simulink model "Final_Model_Project3"  (R2023b)
settings: Solver=ode23tb  StartTime=0.0  StopTime=2.0  MaxStep=1e-5  RelTol=1e-5  AbsTol=1e-5
values from neighbouring files (symbols this model uses):
  alpha_beta = [1 (-1/2) (-1/2); 0 (sqrt(3)/2) (-sqrt(3)/2)]    [Project3.m]
  DC_Link_Cap = 44571.853e-06    (= 0.044571853)    [Project3.m]
  DC_Link_Res = 30e-03    (= 0.03)    [Project3.m]
  F_sampg = 10000    [Project3.m]
  F_swg = 2040    [Project3.m]
  Fc = 100    [Project3.m]
  Fc1 = 500    [Project3.m]
  Fc2 = 10    [Project3.m]
  Fg = 60    [Project3.m]
  Grid_Filter_Ind = 0.12629e-03    (= 0.00012629)    [Project3.m]
  Grid_Filter_Res = 1.19025e-03    (= 0.00119025)    [Project3.m]
  Grid_Line_RMS_Voltage = 690    [Project3.m]
  I_peak = sqrt(2)*Current_base    [Project3.m]
  L_base_pu = 0.2    [Project3.m]
  P_outapp = 2.00e+06    (= 2000000)    [Project3.m]
  Ref_DC_Voltage = 1220    [Project3.m]
  Ts = 1/F_sampg    (= 0.0001)    [Project3.m]
  V_peak = sqrt(2)*Voltage_base    [Project3.m]
  Voltage_Battery = 1259    [Project3.m]
  w_base_pu = 1    [Project3.m]
libraries: spsVoltageMeasurementLib x5, slpidlib x3, spsSeriesRLCBranchLib x2, simulink x2, spsDCVoltageSourceLib x1, simulink_extras x1, spsThreePhaseSeriesRLCBranchLib x1, spsUniversalBridgeLib x1, spsGroundLib x1, spsThreePhaseProgrammableVoltageSourceLib x1, spsThreePhaseVIMeasurementLib x1, sps_lib x1
settings Model: Creator=priya  LastModifiedBy=priya
settings DataIOCC: ReturnWorkspaceOutputs=off

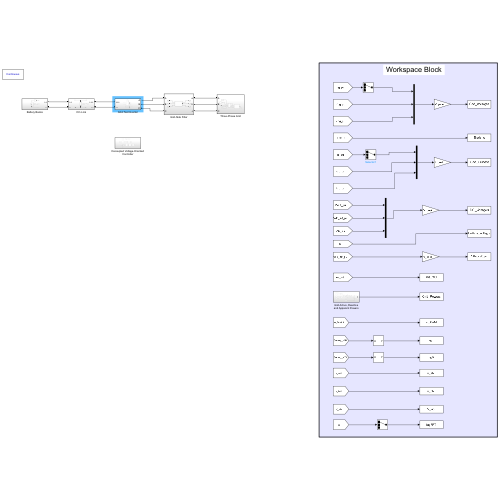
[thumbnail: Simulink's stored preview of the top-level diagram]
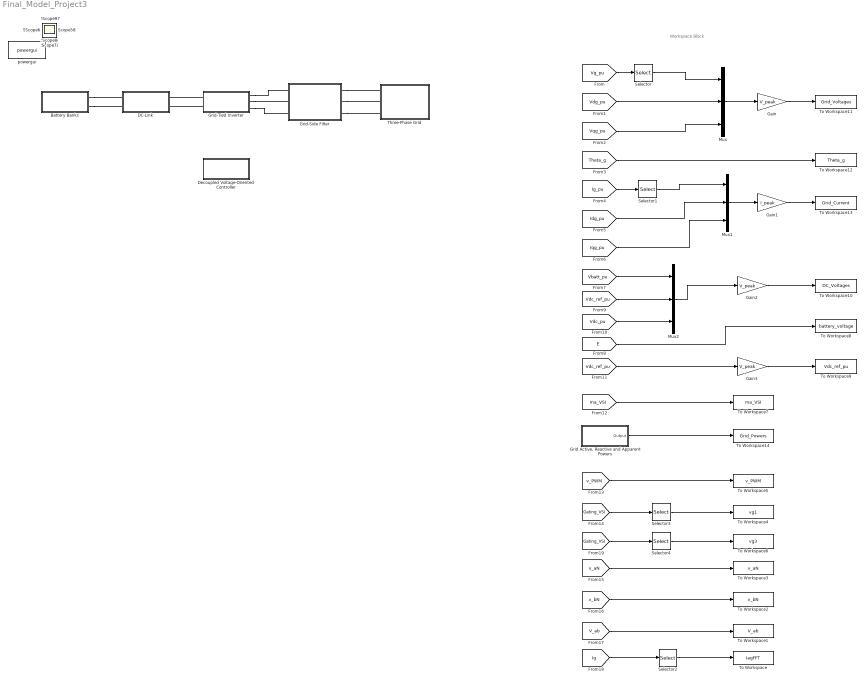
== system Final_Model_Project3 ==
  note: Workspace Block
  Battery Banks : Subsystem
  DC-Link : Subsystem
  Decoupled Voltage-Oriented Controller : Subsystem
  Gain : Gain  Gain=V_peak
  Gain1 : Gain  Gain=I_peak
  Gain2 : Gain  Gain=V_peak
  Gain3 : Gain  Gain=V_peak
  "Grid Active, Reactive and Apparent Powers" : Subsystem
  Grid-Side Filter : Subsystem
  Grid-Tied Inverter : Subsystem
  Mux : Mux  Inputs=3
  Mux1 : Mux  Inputs=3
  Mux2 : Mux  Inputs=3
  Selector : Selector  InputPortWidth=3  IndexOptions=Index vector (dialog)  Indices=[1]  OutputSizes=1
  Selector1 : Selector  InputPortWidth=3  IndexOptions=Index vector (dialog)  Indices=[1]  OutputSizes=1
  Selector2 : Selector  InputPortWidth=3  IndexOptions=Index vector (dialog)  Indices=[1]  OutputSizes=1
  Selector3 : Selector  InputPortWidth=6  IndexOptions=Starting index (dialog)  Indices=[1]  OutputSizes=1
  Selector4 : Selector  InputPortWidth=6  IndexOptions=Starting index (dialog)  Indices=[3]  OutputSizes=1
  Three-Phase Grid : Subsystem
  To Workspace : ToWorkspace  VariableName=IagFFT  SaveFormat=Structure With Time  SampleTime=-1
  To Workspace1 : ToWorkspace  VariableName=V_ab  SampleTime=-1
  To Workspace10 : ToWorkspace  VariableName=DC_Voltages  SampleTime=-1
  To Workspace11 : ToWorkspace  VariableName=Grid_Voltages  SampleTime=-1
  To Workspace12 : ToWorkspace  VariableName=Theta_g  SampleTime=-1
  To Workspace13 : ToWorkspace  VariableName=Grid_Current  SampleTime=-1
  To Workspace14 : ToWorkspace  VariableName=Grid_Powers  SampleTime=-1
  To Workspace2 : ToWorkspace  VariableName=v_bN  SampleTime=-1
  To Workspace3 : ToWorkspace  VariableName=v_aN  SampleTime=-1
  To Workspace4 : ToWorkspace  VariableName=vg1  SampleTime=-1
  To Workspace5 : ToWorkspace  VariableName=v_PWM  SampleTime=-1
  To Workspace6 : ToWorkspace  VariableName=vg3  SampleTime=-1
  To Workspace7 : ToWorkspace  VariableName=ma_VSI  SampleTime=-1
  To Workspace8 : ToWorkspace  VariableName=battery_voltage  SampleTime=-1
  To Workspace9 : ToWorkspace  VariableName=Vdc_ref_pu  SampleTime=-1
  powergui : sps_lib/powergui  Priority=1  SimulationMode=Continuous  SampleTime=50e-6  frequency=60  Iterations=50  frequencyindice=60  Pbase=100e6  ErrMax=1e-4  UnitsV=kV  UnitsW=MW  buscounter=0  FunctionMessages=off  echomessages=off  EnableUseOfTLC=off  CurrentSourceSwitches=off  DisableSnubberDevices=off  DisableRonSwitches=off  DisableVfSwitches=off  DisplayEquations=off  AutomaticDiscreteSolvers=off  SolverType=Tustin/Backward Euler (TBE)  Interpol=off  ExternalGateDelay=off  methode=off  Ts=100  x0status=blocks  SPID=on  SwTol=0  HookPort=off  NonlinearTolerance=1e-4  nMaxIteration=100  ContinueOnMaxIteration=off  RestoreLinks=warning  ResistiveCurrentMeasurement=off  Frange=[0:2:500]  Ylog=off  Xlog=on  ShowGrid=off  save=off  variable=ZData  structure=0  ZoomFFT=off  StartTime=0.0  cycles=1  DisplayStyle=1  fundamental=60  FreqAxis=off  MaxFrequency=1000  frequencyindicesteady=1  RmsSteady=1  display=off
  Scope{,1..10,14..19} (17 alike) : Scope
  wires:
  [Vg_pu] -> Selector/1
  [Ig_pu] -> Selector1/1
  Selector/1 -> Mux/1
  [Vdg_pu] -> Mux/2
  [Vqg_pu] -> Mux/3
  Selector1/1 -> Mux1/1
  [Idg_pu] -> Mux1/2
  [Iqg_pu] -> Mux1/3
  Mux/1 -> Gain/1
  Mux1/1 -> Gain1/1
  [E] -> To Workspace8/1
  [Vbatt_pu] -> Mux2/1
  [Vdc_ref_pu] -> Mux2/2
  [Vdc_pu] -> Mux2/3
  Mux2/1 -> Gain2/1
  [Vdc_ref_pu] -> Gain3/1
  [Ig] -> Selector2/1
  Selector2/1 -> To Workspace/1
  [V_ab] -> To Workspace1/1
  [v_bN] -> To Workspace2/1
  [v_aN] -> To Workspace3/1
  [v_PWM] -> To Workspace5/1
  [Gating_VSI] -> Selector3/1
  Selector3/1 -> To Workspace4/1
  [Gating_VSI] -> Selector4/1
  Selector4/1 -> To Workspace6/1
  [ma_VSI] -> To Workspace7/1
  Gain3/1 -> To Workspace9/1
  Gain2/1 -> To Workspace10/1
  Gain/1 -> To Workspace11/1
  [Theta_g] -> To Workspace12/1
  Gain1/1 -> To Workspace13/1
  "Grid Active, Reactive and Apparent Powers"/1(Output) -> To Workspace14/1
  connections:
  Battery Banks/LConn1 -- DC-Link/LConn1
  Battery Banks/LConn2 -- DC-Link/LConn2
  Grid-Side Filter/RConn1 -- Three-Phase Grid/LConn1
  Grid-Side Filter/RConn2 -- Three-Phase Grid/LConn2
  Grid-Side Filter/RConn3 -- Three-Phase Grid/LConn3
  Grid-Tied Inverter/LConn1 -- DC-Link/RConn1
  Grid-Tied Inverter/LConn2 -- DC-Link/RConn2
  Grid-Tied Inverter/RConn1 -- Grid-Side Filter/LConn1
  Grid-Tied Inverter/RConn2 -- Grid-Side Filter/LConn2
  Grid-Tied Inverter/RConn3 -- Grid-Side Filter/LConn3

== system Final_Model_Project3/Battery Banks ==
  DC Voltage Source : spsDCVoltageSourceLib/DC Voltage Source  Amplitude=Voltage_Battery  Measurements=None
  Series RLC Branch : spsSeriesRLCBranchLib/Series RLC Branch  LConnTagsString=__new0  RConnTagsString=__new0  BranchType=R  Resistance=DC_Link_Res  Inductance=1e-3  SetiL0=off  InitialCurrent=0  Capacitance=1e-6  Setx0=off  InitialVoltage=0  Measurements=None
  Voltage Measurement : spsVoltageMeasurementLib/Voltage Measurement  PhasorSimulation=off  OutputType=Complex  PSBequivalent=0
  ++ : PMIOPort  Side=Left
  -- : PMIOPort  Port=2  Side=Left
  tag scope: E=global
  wires:
  Voltage Measurement/1 -> [E]
  connections:
  --/RConn1 -- Voltage Measurement/LConn2 -- DC Voltage Source/LConn1
  Voltage Measurement/LConn1 -- Series RLC Branch/LConn1 -- DC Voltage Source/RConn1
  Series RLC Branch/RConn1 -- ++/RConn1

== system Final_Model_Project3/DC-Link ==
  Cdc : spsSeriesRLCBranchLib/Series RLC Branch  LConnTagsString=__new0  RConnTagsString=__new0  BranchType=C  Resistance=1  Inductance=1e-3  SetiL0=off  InitialCurrent=0  Capacitance=DC_Link_Cap  Setx0=on  InitialVoltage=2*Ref_DC_Voltage  Measurements=None
  Voltage Measurement : spsVoltageMeasurementLib/Voltage Measurement  PhasorSimulation=off  OutputType=Complex  PSBequivalent=0
  ++ : PMIOPort  Side=Left
  -- : PMIOPort  Port=2  Side=Left
  +++ : PMIOPort  Port=3  Side=Right
  --- : PMIOPort  Port=4  Side=Right
  tag scope: Vdc=global
  wires:
  Voltage Measurement/1 -> [Vdc]
  connections:
  Cdc/LConn1 -- Voltage Measurement/LConn1 -- ++/RConn1 -- +++/RConn1
  Cdc/RConn1 -- Voltage Measurement/LConn2 -- --/RConn1 -- ---/RConn1

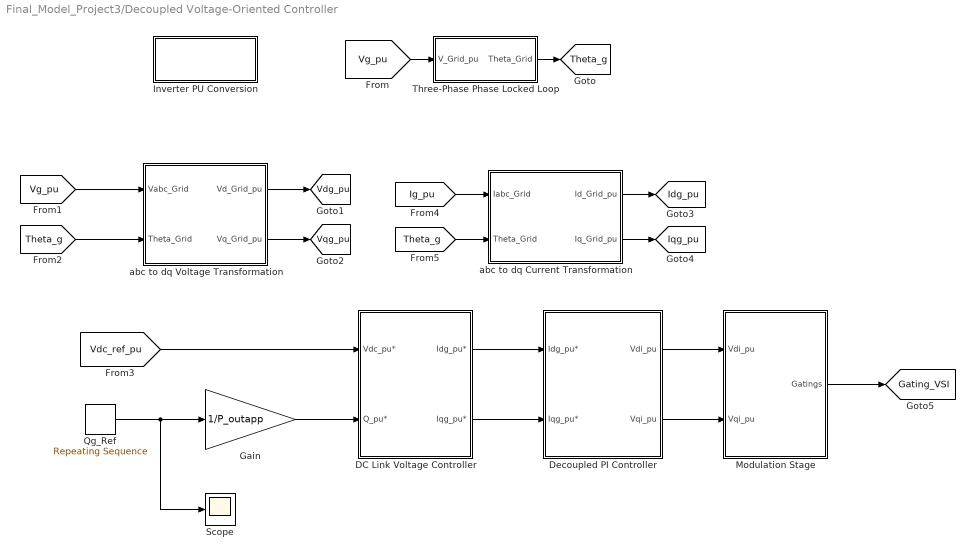
== system Final_Model_Project3/Decoupled Voltage-Oriented Controller ==
  DC Link Voltage Controller : Subsystem
  Decoupled PI Controller : Subsystem
  Gain : Gain  Gain=1/P_outapp
  Inverter PU Conversion : Subsystem
  Modulation Stage : Subsystem
  Qg_Ref : simulink/Sources/Repeating Sequence  rep_seq_t=[0 0.4 0.6 0.8 1 1.2 1.4 1.6 1.8 2]  rep_seq_y=[0 0 1.2e6 1.2e6 0 0 -0.7749e6 -0.7749e6 0 0]
  Scope : Scope
  Three-Phase Phase Locked Loop : Subsystem
  abc to dq Current Transformation : Subsystem
  abc to dq Voltage Transformation : Subsystem
  tag scope: Gating_VSI=global, Idg_pu=global, Iqg_pu=global, Theta_g=global, Vdg_pu=global, Vqg_pu=global
  wires:
  [Vg_pu] -> Three-Phase Phase Locked Loop/1(V_Grid_pu)
  Three-Phase Phase Locked Loop/1(Theta_Grid) -> [Theta_g]
  [Vg_pu] -> abc to dq Voltage Transformation/1(Vabc_Grid)
  [Theta_g] -> abc to dq Voltage Transformation/2(Theta_Grid)
  abc to dq Voltage Transformation/1(Vd_Grid_pu) -> [Vdg_pu]
  abc to dq Voltage Transformation/2(Vq_Grid_pu) -> [Vqg_pu]
  Qg_Ref/1 -> Scope/1, Gain/1
  [Vdc_ref_pu] -> DC Link Voltage Controller/1(Vdc_pu*)
  Gain/1 -> DC Link Voltage Controller/2(Q_pu*)
  [Ig_pu] -> abc to dq Current Transformation/1(Iabc_Grid)
  [Theta_g] -> abc to dq Current Transformation/2(Theta_Grid)
  abc to dq Current Transformation/1(Id_Grid_pu) -> [Idg_pu]
  abc to dq Current Transformation/2(Iq_Grid_pu) -> [Iqg_pu]
  DC Link Voltage Controller/1(Idg_pu*) -> Decoupled PI Controller/1(Idg_pu*)
  DC Link Voltage Controller/2(Iqg_pu*) -> Decoupled PI Controller/2(Iqg_pu*)
  Decoupled PI Controller/1(Vdi_pu) -> Modulation Stage/1(Vdi_pu)
  Decoupled PI Controller/2(Vqi_pu) -> Modulation Stage/2(Vqi_pu)
  Modulation Stage/1(Gatings) -> [Gating_VSI]

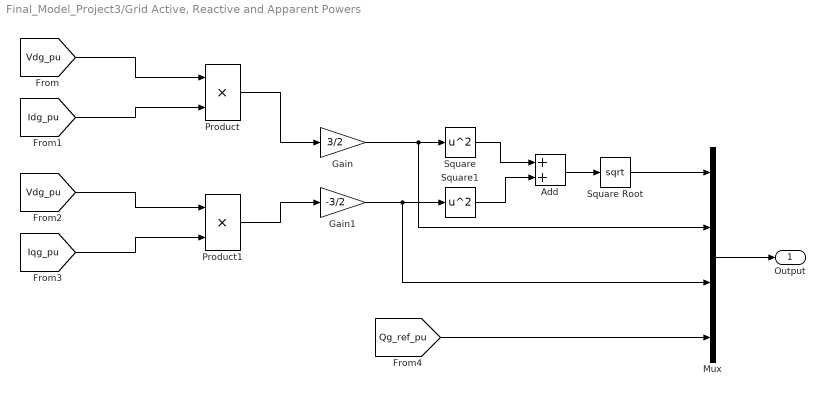
== system Final_Model_Project3/Grid Active, Reactive and Apparent Powers ==
  Add : Sum
  Gain : Gain  Gain=3/2
  Gain1 : Gain  Gain=-3/2
  Mux : Mux
  Product : Product
  Product1 : Product
  Square : Math  Operator=square
  Square Root : Sqrt
  Square1 : Math  Operator=square
  Output : Outport
  wires:
  [Vdg_pu] -> Product/1
  [Idg_pu] -> Product/2
  Product/1 -> Gain/1
  [Vdg_pu] -> Product1/1
  [Iqg_pu] -> Product1/2
  Product1/1 -> Gain1/1
  Gain/1 -> Mux/2, Square/1
  Gain1/1 -> Mux/3, Square1/1
  Square/1 -> Add/1
  Square1/1 -> Add/2
  Add/1 -> Square Root/1
  Square Root/1 -> Mux/1
  [Qg_ref_pu] -> Mux/4
  Mux/1 -> Output/1

== system Final_Model_Project3/Grid-Side Filter ==
  Three-Phase Series RLC Branch : spsThreePhaseSeriesRLCBranchLib/Three-Phase Series RLC Branch  LConnTagsString=A|B|C  RConnTagsString=A|B|C  BranchType=RL  Resistance=Grid_Filter_Res  Inductance=Grid_Filter_Ind  Capacitance=1e-6  Measurements=None
  A : PMIOPort  Side=Left
  B : PMIOPort  Port=2  Side=Left
  C : PMIOPort  Port=3  Side=Left
  a : PMIOPort  Port=4  Side=Right
  b : PMIOPort  Port=5  Side=Right
  c : PMIOPort  Port=6  Side=Right
  connections:
  Three-Phase Series RLC Branch/LConn1 -- a/RConn1
  Three-Phase Series RLC Branch/LConn2 -- b/RConn1
  c/RConn1 -- Three-Phase Series RLC Branch/LConn3
  A/RConn1 -- Three-Phase Series RLC Branch/RConn1
  B/RConn1 -- Three-Phase Series RLC Branch/RConn2
  C/RConn1 -- Three-Phase Series RLC Branch/RConn3

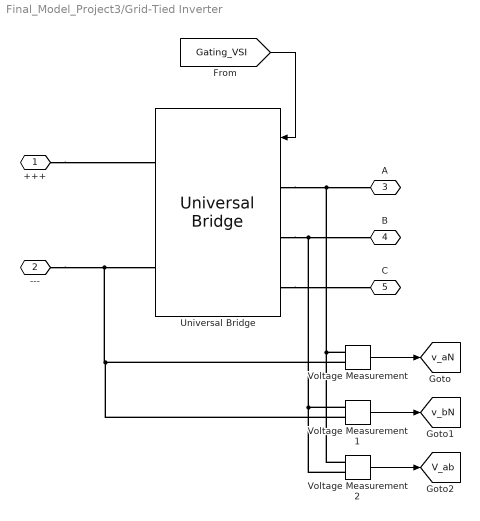
== system Final_Model_Project3/Grid-Tied Inverter ==
  Universal Bridge : spsUniversalBridgeLib/Universal Bridge  Arms=3  SnubberResistance=1e5  SnubberCapacitance=inf  Device=IGBT / Diodes  Ron=1e-6  Lon=0  ForwardVoltages="[  0  0  ]"  ForwardVoltage=0  GTOparameters=[ 10e-6 , 20e-6 ]  IGBTparameters=[ 1e-6 , 2e-6 ]  Measurements=None  Measurements_2=None  converterType=Rectifier
  Voltage Measurement : spsVoltageMeasurementLib/Voltage Measurement  PhasorSimulation=off  OutputType=Complex  PSBequivalent=0
  Voltage Measurement1 : spsVoltageMeasurementLib/Voltage Measurement  PhasorSimulation=off  OutputType=Complex  PSBequivalent=0
  Voltage Measurement2 : spsVoltageMeasurementLib/Voltage Measurement  PhasorSimulation=off  OutputType=Complex  PSBequivalent=0
  +++ : PMIOPort  Side=Left
  --- : PMIOPort  Port=2  Side=Left
  A : PMIOPort  Port=3  Side=Right
  B : PMIOPort  Port=4  Side=Right
  C : PMIOPort  Port=5  Side=Right
  tag scope: V_ab=global, v_aN=global, v_bN=global
  wires:
  [Gating_VSI] -> Universal Bridge/1
  Voltage Measurement/1 -> [v_aN]
  Voltage Measurement1/1 -> [v_bN]
  Voltage Measurement2/1 -> [V_ab]
  connections:
  +++/RConn1 -- Universal Bridge/RConn1
  ---/RConn1 -- Voltage Measurement1/LConn2 -- Voltage Measurement/LConn2 -- Universal Bridge/RConn2
  Universal Bridge/LConn1 -- Voltage Measurement2/LConn1 -- Voltage Measurement/LConn1 -- A/RConn1
  Universal Bridge/LConn2 -- Voltage Measurement2/LConn2 -- Voltage Measurement1/LConn1 -- B/RConn1
  Universal Bridge/LConn3 -- C/RConn1

== system Final_Model_Project3/Three-Phase Grid ==
  Ground : spsGroundLib/Ground  LConnTagsString=a
  Three-Phase Programmable Voltage Source : spsThreePhaseProgrammableVoltageSourceLib/Three-Phase Programmable Voltage Source  PositiveSequence=[Grid_Line_RMS_Voltage 0 Fg]  VariationEntity=None  VariationType=Table of time-amplitude pairs  VariationTypeAlt=Step  VariationStep=0.5  VariationRate=10  VariationMagnitude=0.3  VariationFrequency=2  VariationTiming=[1 2]  VariationPhaseA=off  Amplitudes=[1 0.8 1.2 1.0]  TimeValues=[0 0.1 0.15 0.2]  HarmonicGeneration=off  HarmonicA=[3 0.2 -25 0]  HarmonicB=[2 0.15 35 2]  Timing="[0.05  3]"  BusType=swing  Pref=0  Qref=0  Qmin=-inf  Qmax=inf
  Three-Phase V-I Measurement : spsThreePhaseVIMeasurementLib/Three-Phase V-I Measurement  VoltageMeasurement=phase-to-ground  SetLabelV=off  LabelV=Vabc  Vpu=off  VpuLL=off  CurrentMeasurement=yes  SetLabelI=off  LabelI=Iabc  Ipu=off  Pbase=100e6  Vbase=500e3  OutputType=Complex  PhasorSimulation=off  PSBequivalent=0
  A : PMIOPort  Side=Left
  B : PMIOPort  Port=2  Side=Left
  C : PMIOPort  Port=3  Side=Left
  tag scope: Ig=global, Vg=global
  wires:
  Three-Phase V-I Measurement/1 -> [Vg]
  Three-Phase V-I Measurement/2 -> [Ig]
  connections:
  Three-Phase Programmable Voltage Source/LConn1 -- Ground/LConn1
  Three-Phase V-I Measurement/LConn1 -- Three-Phase Programmable Voltage Source/RConn1
  Three-Phase V-I Measurement/LConn2 -- Three-Phase Programmable Voltage Source/RConn2
  Three-Phase V-I Measurement/LConn3 -- Three-Phase Programmable Voltage Source/RConn3
  Three-Phase V-I Measurement/RConn1 -- A/RConn1
  Three-Phase V-I Measurement/RConn2 -- B/RConn1
  Three-Phase V-I Measurement/RConn3 -- C/RConn1

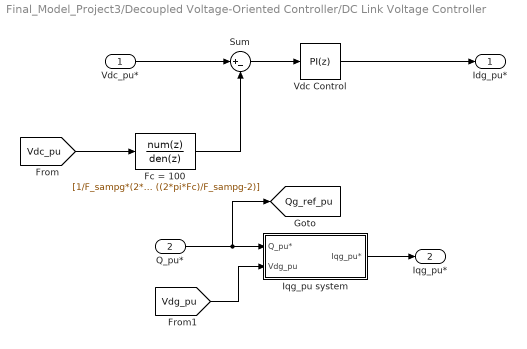
== system Final_Model_Project3/Decoupled Voltage-Oriented Controller/DC Link Voltage Controller ==
  Vdc_pu* : Inport
  Q_pu* : Inport  Port=2
  Fc = 100 : DiscreteTransferFcn  Numerator=[1/F_sampg*(2*pi*Fc) 1/F_sampg*(2*pi*Fc)]  Denominator=[((2*pi*Fc)/F_sampg+2) ((2*pi*Fc)/F_sampg-2)]  SampleTime=Ts
  Iqg_pu system : Subsystem
  Sum : Sum  Inputs=|+-
  Vdc Control : slpidlib/PID Controller  Controller=PI  Form=Parallel  TimeDomain=Discrete-time  UseExternalTs=off  SampleTime=Ts  IntegratorMethod=Forward Euler  FilterMethod=Forward Euler  ControllerParametersSource=internal  P=1  I=200  UseKiTs=off  D=0  N=100  UseFilter=on  TunerSelectOption=Transfer Function Based (PID Tuner App)  InitialConditionSource=internal  InitialConditionForIntegrator=0  InitialConditionForFilter=0  DifferentiatorICPrevScaledInput=0  ExternalReset=none  TrackingMode=off  Kt=1  LimitOutput=on  SatLimitsSource=internal  UpperSaturationLimit=1.5  LowerSaturationLimit=-1.5  LinearizeAsGain=on  AntiWindupMode=none  Kb=1  LimitIntegrator=off  UpperIntegratorSaturationLimit=inf  LowerIntegratorSaturationLimit=-inf  POutMin=[]  POutMax=[]  IOutMin=[]  IOutMax=[]  DOutMin=[]  DOutMax=[]  NOutMin=[]  NOutMax=[]  SumOutMin=[]  SumOutMax=[]  SaturationOutMin=[]  SaturationOutMax=[]  PParamMin=[]  PParamMax=[]  IParamMin=[]  IParamMax=[]  DParamMin=[]  DParamMax=[]  NParamMin=[]  NParamMax=[]  KbParamMin=[]  KbParamMax=[]  KtParamMin=[]  KtParamMax=[]  KbOutMin=[]  KbOutMax=[]  KtOutMin=[]  KtOutMax=[]  IntegratorOutMin=[]  IntegratorOutMax=[]  FilterOutMin=[]  FilterOutMax=[]  SumI1OutMin=[]  SumI1OutMax=[]  SumI2OutMin=[]  SumI2OutMax=[]  SumI3OutMin=[]  SumI3OutMax=[]  SumI4OutMin=[]  SumI4OutMax=[]  SumDOutMin=[]  SumDOutMax=[]  DifferentiatorOutMin=[]  DifferentiatorOutMax=[]  FilterDiffOutCoefMin=[]  FilterDiffOutCoefMax=[]  ReciprocalOutMin=[]  ReciprocalOutMax=[]  SumDenOutMin=[]  SumDenOutMax=[]  SumNumOutMin=[]  SumNumOutMax=[]  DivideOutMin=[]  DivideOutMax=[]  UdiffTsProdOutMin=[]  UdiffTsProdOutMax=[]  NTsProdOutMin=[]  NTsProdOutMax=[]  UintegralTsProdOutMin=[]  UintegralTsProdOutMax=[]  UngainTsProdOutMin=[]  UngainTsProdOutMax=[]  ClampingZeroOutDataTypeStr=Inherit: Inherit via back propagation  ClampingZeroOutMin=[]  ClampingZeroOutMax=[]  FilterDenConstantOutDataTypeStr=Inherit: Inherit via back propagation  FilterDenConstantOutMin=[]  FilterDenConstantOutMax=[]  PCopyOutDataTypeStr=Inherit: Inherit via back propagation  PCopyOutMin=[]  PCopyOutMax=[]  NCopyOutDataTypeStr=Inherit: Inherit via back propagation  NCopyOutMin=[]  NCopyOutMax=[]  IntegratorContinuousStateAttributes=''  IntegratorStateMustResolveToSignalObject=off  IntegratorRTWStateStorageClass=Auto  FilterContinuousStateAttributes=''  FilterStateMustResolveToSignalObject=off  FilterRTWStateStorageClass=Auto  ParallelPVariant=InternalParameters  IdealPVariant=Disabled  IVariant=InternalParameters  DVariant=Disabled  IntegratorVariant=Discrete  SatVariant=Enabled  AWVariant=Passthrough  PCopyVariant=Disabled  TRVariant=Disabled  FdbkBlocksVariant=Forward  IdealPFdbkVariant=Disabled  SatFdbkVariant=Disabled  DerivativeFilterVariant=Disabled  NVariant=Disabled  NCopyVariant=Disabled_SignalSpec  FilterICVariant=Disabled  IntegratorICVariant=InternalICs  ExternalResetVariant=Disabled  TRSumVariant=Passthrough  SumFdbkVariant=Disabled  SumVariant=Sum_PI  TsampFilterVariant=InternalTs  TsampNgainVariant=Passthrough  TsampIntegralVariant=Disabled_SignalSpec  ExternalSaturationOutDataTypeStr=Inherit: Same as second input
  Idg_pu* : Outport
  Iqg_pu* : Outport  Port=2
  tag scope: Qg_ref_pu=global
  wires:
  Vdc_pu*/1 -> Sum/1
  Fc = 100/1 -> Sum/2
  Q_pu*/1 -> [Qg_ref_pu], Iqg_pu system/1(Q_pu*)
  [Vdg_pu] -> Iqg_pu system/2(Vdg_pu)
  Iqg_pu system/1(Iqg_pu*) -> Iqg_pu*/1
  [Vdc_pu] -> Fc = 100/1
  Sum/1 -> Vdc Control/1
  Vdc Control/1 -> Idg_pu*/1

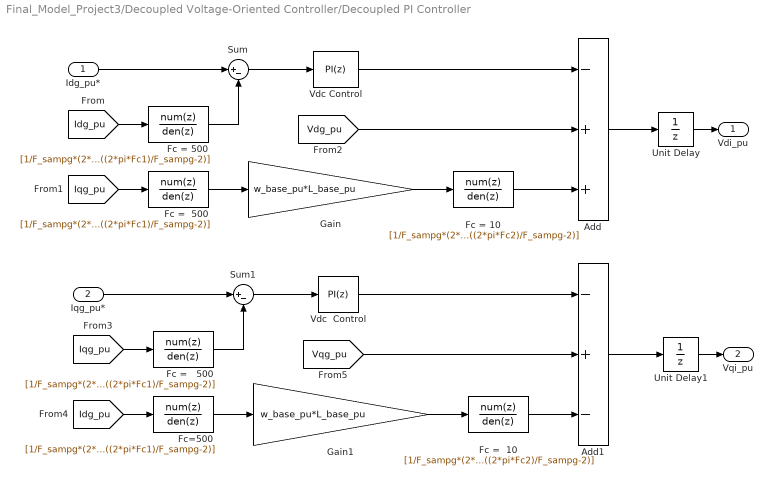
== system Final_Model_Project3/Decoupled Voltage-Oriented Controller/Decoupled PI Controller ==
  Idg_pu* : Inport
  Iqg_pu* : Inport  Port=2
  Add : Sum  Inputs=-++
  Add1 : Sum  Inputs=-+-
  Fc =   500 : DiscreteTransferFcn  Numerator=[1/F_sampg*(2*pi*Fc1) 1/F_sampg*(2*pi*Fc1)]  Denominator=[((2*pi*Fc1)/F_sampg+2) ((2*pi*Fc1)/F_sampg-2)]  SampleTime=Ts
  Fc =  10 : DiscreteTransferFcn  Numerator=[1/F_sampg*(2*pi*Fc2) 1/F_sampg*(2*pi*Fc2)]  Denominator=[((2*pi*Fc2)/F_sampg+2) ((2*pi*Fc2)/F_sampg-2)]  SampleTime=Ts
  Fc =  500 : DiscreteTransferFcn  Numerator=[1/F_sampg*(2*pi*Fc1) 1/F_sampg*(2*pi*Fc1)]  Denominator=[((2*pi*Fc1)/F_sampg+2) ((2*pi*Fc1)/F_sampg-2)]  SampleTime=Ts
  Fc = 10 : DiscreteTransferFcn  Numerator=[1/F_sampg*(2*pi*Fc2) 1/F_sampg*(2*pi*Fc2)]  Denominator=[((2*pi*Fc2)/F_sampg+2) ((2*pi*Fc2)/F_sampg-2)]  SampleTime=Ts
  Fc = 500 : DiscreteTransferFcn  Numerator=[1/F_sampg*(2*pi*Fc1) 1/F_sampg*(2*pi*Fc1)]  Denominator=[((2*pi*Fc1)/F_sampg+2) ((2*pi*Fc1)/F_sampg-2)]  SampleTime=Ts
  Fc=500 : DiscreteTransferFcn  Numerator=[1/F_sampg*(2*pi*Fc1) 1/F_sampg*(2*pi*Fc1)]  Denominator=[((2*pi*Fc1)/F_sampg+2) ((2*pi*Fc1)/F_sampg-2)]  SampleTime=Ts
  Gain : Gain  Gain=w_base_pu*L_base_pu
  Gain1 : Gain  Gain=w_base_pu*L_base_pu
  Sum : Sum  Inputs=|+-
  Sum1 : Sum  Inputs=|+-
  Unit Delay : UnitDelay  SampleTime=Ts  HasFrameUpgradeWarning=on
  Unit Delay1 : UnitDelay  SampleTime=Ts  HasFrameUpgradeWarning=on
  Vdc  Control : slpidlib/PID Controller  Controller=PI  Form=Parallel  TimeDomain=Discrete-time  UseExternalTs=off  SampleTime=Ts  IntegratorMethod=Forward Euler  FilterMethod=Forward Euler  ControllerParametersSource=internal  P=0.3  I=200  UseKiTs=off  D=0  N=100  UseFilter=on  TunerSelectOption=Transfer Function Based (PID Tuner App)  InitialConditionSource=internal  InitialConditionForIntegrator=0  InitialConditionForFilter=0  DifferentiatorICPrevScaledInput=0  ExternalReset=none  TrackingMode=off  Kt=1  LimitOutput=on  SatLimitsSource=internal  UpperSaturationLimit=1.0  LowerSaturationLimit=-1.0  LinearizeAsGain=on  AntiWindupMode=none  Kb=1  LimitIntegrator=off  UpperIntegratorSaturationLimit=inf  LowerIntegratorSaturationLimit=-inf  POutMin=[]  POutMax=[]  IOutMin=[]  IOutMax=[]  DOutMin=[]  DOutMax=[]  NOutMin=[]  NOutMax=[]  SumOutMin=[]  SumOutMax=[]  SaturationOutMin=[]  SaturationOutMax=[]  PParamMin=[]  PParamMax=[]  IParamMin=[]  IParamMax=[]  DParamMin=[]  DParamMax=[]  NParamMin=[]  NParamMax=[]  KbParamMin=[]  KbParamMax=[]  KtParamMin=[]  KtParamMax=[]  KbOutMin=[]  KbOutMax=[]  KtOutMin=[]  KtOutMax=[]  IntegratorOutMin=[]  IntegratorOutMax=[]  FilterOutMin=[]  FilterOutMax=[]  SumI1OutMin=[]  SumI1OutMax=[]  SumI2OutMin=[]  SumI2OutMax=[]  SumI3OutMin=[]  SumI3OutMax=[]  SumI4OutMin=[]  SumI4OutMax=[]  SumDOutMin=[]  SumDOutMax=[]  DifferentiatorOutMin=[]  DifferentiatorOutMax=[]  FilterDiffOutCoefMin=[]  FilterDiffOutCoefMax=[]  ReciprocalOutMin=[]  ReciprocalOutMax=[]  SumDenOutMin=[]  SumDenOutMax=[]  SumNumOutMin=[]  SumNumOutMax=[]  DivideOutMin=[]  DivideOutMax=[]  UdiffTsProdOutMin=[]  UdiffTsProdOutMax=[]  NTsProdOutMin=[]  NTsProdOutMax=[]  UintegralTsProdOutMin=[]  UintegralTsProdOutMax=[]  UngainTsProdOutMin=[]  UngainTsProdOutMax=[]  ClampingZeroOutDataTypeStr=Inherit: Inherit via back propagation  ClampingZeroOutMin=[]  ClampingZeroOutMax=[]  FilterDenConstantOutDataTypeStr=Inherit: Inherit via back propagation  FilterDenConstantOutMin=[]  FilterDenConstantOutMax=[]  PCopyOutDataTypeStr=Inherit: Inherit via back propagation  PCopyOutMin=[]  PCopyOutMax=[]  NCopyOutDataTypeStr=Inherit: Inherit via back propagation  NCopyOutMin=[]  NCopyOutMax=[]  IntegratorContinuousStateAttributes=''  IntegratorStateMustResolveToSignalObject=off  IntegratorRTWStateStorageClass=Auto  FilterContinuousStateAttributes=''  FilterStateMustResolveToSignalObject=off  FilterRTWStateStorageClass=Auto  ParallelPVariant=InternalParameters  IdealPVariant=Disabled  IVariant=InternalParameters  DVariant=Disabled  IntegratorVariant=Discrete  SatVariant=Enabled  AWVariant=Passthrough  PCopyVariant=Disabled  TRVariant=Disabled  FdbkBlocksVariant=Forward  IdealPFdbkVariant=Disabled  SatFdbkVariant=Disabled  DerivativeFilterVariant=Disabled  NVariant=Disabled  NCopyVariant=Disabled_SignalSpec  FilterICVariant=Disabled  IntegratorICVariant=InternalICs  ExternalResetVariant=Disabled  TRSumVariant=Passthrough  SumFdbkVariant=Disabled  SumVariant=Sum_PI  TsampFilterVariant=InternalTs  TsampNgainVariant=Passthrough  TsampIntegralVariant=Disabled_SignalSpec  ExternalSaturationOutDataTypeStr=Inherit: Same as second input
  Vdc Control : slpidlib/PID Controller  Controller=PI  Form=Parallel  TimeDomain=Discrete-time  UseExternalTs=off  SampleTime=Ts  IntegratorMethod=Forward Euler  FilterMethod=Forward Euler  ControllerParametersSource=internal  P=0.3  I=200  UseKiTs=off  D=0  N=100  UseFilter=on  TunerSelectOption=Transfer Function Based (PID Tuner App)  InitialConditionSource=internal  InitialConditionForIntegrator=0  InitialConditionForFilter=0  DifferentiatorICPrevScaledInput=0  ExternalReset=none  TrackingMode=off  Kt=1  LimitOutput=on  SatLimitsSource=internal  UpperSaturationLimit=1.0  LowerSaturationLimit=-1.0  LinearizeAsGain=on  AntiWindupMode=none  Kb=1  LimitIntegrator=off  UpperIntegratorSaturationLimit=inf  LowerIntegratorSaturationLimit=-inf  POutMin=[]  POutMax=[]  IOutMin=[]  IOutMax=[]  DOutMin=[]  DOutMax=[]  NOutMin=[]  NOutMax=[]  SumOutMin=[]  SumOutMax=[]  SaturationOutMin=[]  SaturationOutMax=[]  PParamMin=[]  PParamMax=[]  IParamMin=[]  IParamMax=[]  DParamMin=[]  DParamMax=[]  NParamMin=[]  NParamMax=[]  KbParamMin=[]  KbParamMax=[]  KtParamMin=[]  KtParamMax=[]  KbOutMin=[]  KbOutMax=[]  KtOutMin=[]  KtOutMax=[]  IntegratorOutMin=[]  IntegratorOutMax=[]  FilterOutMin=[]  FilterOutMax=[]  SumI1OutMin=[]  SumI1OutMax=[]  SumI2OutMin=[]  SumI2OutMax=[]  SumI3OutMin=[]  SumI3OutMax=[]  SumI4OutMin=[]  SumI4OutMax=[]  SumDOutMin=[]  SumDOutMax=[]  DifferentiatorOutMin=[]  DifferentiatorOutMax=[]  FilterDiffOutCoefMin=[]  FilterDiffOutCoefMax=[]  ReciprocalOutMin=[]  ReciprocalOutMax=[]  SumDenOutMin=[]  SumDenOutMax=[]  SumNumOutMin=[]  SumNumOutMax=[]  DivideOutMin=[]  DivideOutMax=[]  UdiffTsProdOutMin=[]  UdiffTsProdOutMax=[]  NTsProdOutMin=[]  NTsProdOutMax=[]  UintegralTsProdOutMin=[]  UintegralTsProdOutMax=[]  UngainTsProdOutMin=[]  UngainTsProdOutMax=[]  ClampingZeroOutDataTypeStr=Inherit: Inherit via back propagation  ClampingZeroOutMin=[]  ClampingZeroOutMax=[]  FilterDenConstantOutDataTypeStr=Inherit: Inherit via back propagation  FilterDenConstantOutMin=[]  FilterDenConstantOutMax=[]  PCopyOutDataTypeStr=Inherit: Inherit via back propagation  PCopyOutMin=[]  PCopyOutMax=[]  NCopyOutDataTypeStr=Inherit: Inherit via back propagation  NCopyOutMin=[]  NCopyOutMax=[]  IntegratorContinuousStateAttributes=''  IntegratorStateMustResolveToSignalObject=off  IntegratorRTWStateStorageClass=Auto  FilterContinuousStateAttributes=''  FilterStateMustResolveToSignalObject=off  FilterRTWStateStorageClass=Auto  ParallelPVariant=InternalParameters  IdealPVariant=Disabled  IVariant=InternalParameters  DVariant=Disabled  IntegratorVariant=Discrete  SatVariant=Enabled  AWVariant=Passthrough  PCopyVariant=Disabled  TRVariant=Disabled  FdbkBlocksVariant=Forward  IdealPFdbkVariant=Disabled  SatFdbkVariant=Disabled  DerivativeFilterVariant=Disabled  NVariant=Disabled  NCopyVariant=Disabled_SignalSpec  FilterICVariant=Disabled  IntegratorICVariant=InternalICs  ExternalResetVariant=Disabled  TRSumVariant=Passthrough  SumFdbkVariant=Disabled  SumVariant=Sum_PI  TsampFilterVariant=InternalTs  TsampNgainVariant=Passthrough  TsampIntegralVariant=Disabled_SignalSpec  ExternalSaturationOutDataTypeStr=Inherit: Same as second input
  Vdi_pu : Outport
  Vqi_pu : Outport  Port=2
  wires:
  [Idg_pu] -> Fc = 500/1
  Fc = 500/1 -> Sum/2
  Idg_pu*/1 -> Sum/1
  Sum/1 -> Vdc Control/1
  Vdc Control/1 -> Add/1
  [Vdg_pu] -> Add/2
  [Iqg_pu] -> Fc =  500/1
  Fc =  500/1 -> Gain/1
  Gain/1 -> Fc = 10/1
  Fc = 10/1 -> Add/3
  Add/1 -> Unit Delay/1
  Unit Delay/1 -> Vdi_pu/1
  [Idg_pu] -> Fc=500/1
  Sum1/1 -> Vdc  Control/1
  Vdc  Control/1 -> Add1/1
  Gain1/1 -> Fc =  10/1
  [Iqg_pu] -> Fc =   500/1
  Fc =   500/1 -> Sum1/2
  Iqg_pu*/1 -> Sum1/1
  Add1/1 -> Unit Delay1/1
  Fc =  10/1 -> Add1/3
  [Vqg_pu] -> Add1/2
  Unit Delay1/1 -> Vqi_pu/1
  Fc=500/1 -> Gain1/1

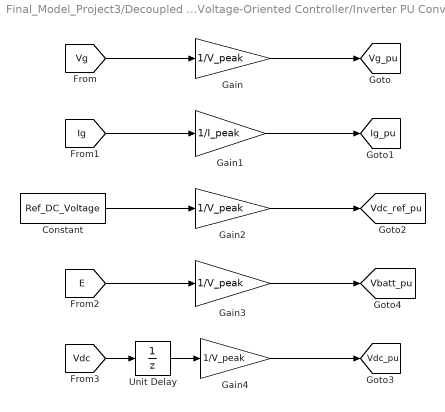
== system Final_Model_Project3/Decoupled Voltage-Oriented Controller/Inverter PU Conversion ==
  Constant : Constant  Value=Ref_DC_Voltage
  Gain{,2..4} (4 alike) : Gain  Gain=1/V_peak
  Gain1 : Gain  Gain=1/I_peak
  Unit Delay : UnitDelay  SampleTime=1/F_sampg  HasFrameUpgradeWarning=on
  tag scope: Ig_pu=global, Vbatt_pu=global, Vdc_pu=global, Vdc_ref_pu=global, Vg_pu=global
  wires:
  [Vg] -> Gain/1
  [Ig] -> Gain1/1
  Constant/1 -> Gain2/1
  [E] -> Gain3/1
  Unit Delay/1 -> Gain4/1
  [Vdc] -> Unit Delay/1
  Gain/1 -> [Vg_pu]
  Gain1/1 -> [Ig_pu]
  Gain2/1 -> [Vdc_ref_pu]
  Gain3/1 -> [Vbatt_pu]
  Gain4/1 -> [Vdc_pu]

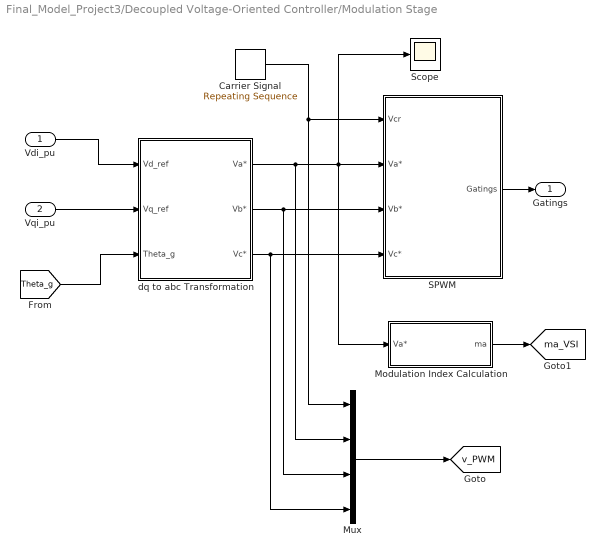
== system Final_Model_Project3/Decoupled Voltage-Oriented Controller/Modulation Stage ==
  Vdi_pu : Inport
  Vqi_pu : Inport  Port=2
  Carrier Signal : simulink/Sources/Repeating Sequence  rep_seq_t=[0 1/(2*F_swg) 1/F_swg]  rep_seq_y=[-1 1 -1]
  Modulation Index Calculation : Subsystem
  Mux : Mux
  SPWM : Subsystem
  Scope : Scope
  dq to abc Transformation : Subsystem
  Gatings : Outport
  tag scope: ma_VSI=global, v_PWM=global
  wires:
  Vqi_pu/1 -> dq to abc Transformation/2(Vq_ref)
  Vdi_pu/1 -> dq to abc Transformation/1(Vd_ref)
  [Theta_g] -> dq to abc Transformation/3(Theta_g)
  SPWM/1(Gatings) -> Gatings/1
  Carrier Signal/1 -> Mux/1, SPWM/1(Vcr)
  dq to abc Transformation/1(Va*) -> Mux/2, Scope/1, Modulation Index Calculation/1(Va*), SPWM/2(Va*)
  dq to abc Transformation/2(Vb*) -> Mux/3, SPWM/3(Vb*)
  dq to abc Transformation/3(Vc*) -> Mux/4, SPWM/4(Vc*)
  Mux/1 -> [v_PWM]
  Modulation Index Calculation/1(ma) -> [ma_VSI]

== system Final_Model_Project3/Decoupled Voltage-Oriented Controller/Three-Phase Phase Locked Loop ==
  V_Grid_pu : Inport
  Alpha - Beta Transformation : Subsystem
  Cartesian to Polar : simulink_extras/Transformations/Cartesian to Polar
  Demux : Demux  Outputs=3
  Unit Delay : UnitDelay  SampleTime=-1  HasFrameUpgradeWarning=on
  Theta_Grid : Outport
  wires:
  V_Grid_pu/1 -> Demux/1
  Demux/2 -> Alpha - Beta Transformation/2(Vbn)
  Demux/1 -> Alpha - Beta Transformation/1(Van)
  Demux/3 -> Alpha - Beta Transformation/3(Vcn)
  Alpha - Beta Transformation/1(V_Alpha) -> Cartesian to Polar/1
  Alpha - Beta Transformation/2(V_Beta) -> Cartesian to Polar/2
  Unit Delay/1 -> Theta_Grid/1
  Cartesian to Polar/2 -> Unit Delay/1

== system Final_Model_Project3/Decoupled Voltage-Oriented Controller/abc to dq Current Transformation ==
  Iabc_Grid : Inport
  Theta_Grid : Inport  Port=2
  Id : Fcn  Expr=(2/3)*(u(1)*cos(u(4)) + u(2)*cos(u(4)-(2*pi/3)) + u(3)*cos(u(4)-(4*pi/3)))
  Iq : Fcn  Expr=(2/3)*(-u(1)*sin(u(4)) - u(2)*sin(u(4)-(2*pi/3)) - u(3)*sin(u(4)-(4*pi/3)))
  Mux : Mux  Inputs=2
  Id_Grid_pu : Outport
  Iq_Grid_pu : Outport  Port=2
  wires:
  Iabc_Grid/1 -> Mux/1
  Theta_Grid/1 -> Mux/2
  Mux/1 -> Iq/1, Id/1
  Iq/1 -> Iq_Grid_pu/1
  Id/1 -> Id_Grid_pu/1

== system Final_Model_Project3/Decoupled Voltage-Oriented Controller/abc to dq Voltage Transformation ==
  Vabc_Grid : Inport
  Theta_Grid : Inport  Port=2
  Mux : Mux  Inputs=2
  Vd : Fcn  Expr=(2/3)*(u(1)*cos(u(4)) + u(2)*cos(u(4)-(2*pi/3)) + u(3)*cos(u(4)-(4*pi/3)))
  Vq : Fcn  Expr=(2/3)*(-u(1)*sin(u(4)) - u(2)*sin(u(4)-(2*pi/3)) - u(3)*sin(u(4)-(4*pi/3)))
  Vd_Grid_pu : Outport
  Vq_Grid_pu : Outport  Port=2
  wires:
  Vabc_Grid/1 -> Mux/1
  Theta_Grid/1 -> Mux/2
  Mux/1 -> Vq/1, Vd/1
  Vd/1 -> Vd_Grid_pu/1
  Vq/1 -> Vq_Grid_pu/1

== system Final_Model_Project3/Decoupled Voltage-Oriented Controller/DC Link Voltage Controller/Iqg_pu system ==
  Q_pu* : Inport
  Vdg_pu : Inport  Port=2
  Divide : Product  Inputs=*/
  Gain : Gain  Gain=-1.5
  Gain1 : Gain  Gain=sqrt(2)
  Iqg_pu* : Outport
  wires:
  Vdg_pu/1 -> Gain/1
  Gain/1 -> Divide/2
  Divide/1 -> Iqg_pu*/1
  Q_pu*/1 -> Gain1/1
  Gain1/1 -> Divide/1

== system Final_Model_Project3/Decoupled Voltage-Oriented Controller/Modulation Stage/Modulation Index Calculation ==
  Va* : Inport
  Gain : Gain  Gain=sqrt(2)
  RMS : Subsystem
  ma : Outport
  wires:
  Va*/1 -> RMS/1(signal)
  RMS/1(rms) -> Gain/1
  Gain/1 -> ma/1

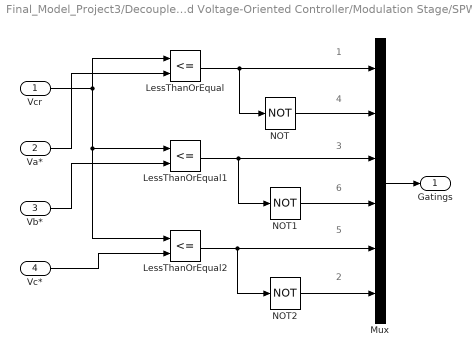
== system Final_Model_Project3/Decoupled Voltage-Oriented Controller/Modulation Stage/SPWM ==
  note: 1
  note: 4
  note: 3
  note: 6
  note: 5
  note: 2
  Vcr : Inport
  Va* : Inport  Port=2
  Vb* : Inport  Port=3
  Vc* : Inport  Port=4
  LessThanOrEqual : RelationalOperator  Operator=<=  OutDataTypeStr=boolean  RndMeth=Simplest  InputSameDT=off
  LessThanOrEqual1 : RelationalOperator  Operator=<=  OutDataTypeStr=boolean  RndMeth=Simplest  InputSameDT=off
  LessThanOrEqual2 : RelationalOperator  Operator=<=  OutDataTypeStr=boolean  RndMeth=Simplest  InputSameDT=off
  Mux : Mux  Inputs=6
  NOT : Logic  Operator=NOT  IconShape=distinctive  AllPortsSameDT=off  OutDataTypeStr=boolean
  NOT1 : Logic  Operator=NOT  IconShape=distinctive  AllPortsSameDT=off  OutDataTypeStr=boolean
  NOT2 : Logic  Operator=NOT  IconShape=distinctive  AllPortsSameDT=off  OutDataTypeStr=boolean
  Gatings : Outport
  wires:
  Vcr/1 -> LessThanOrEqual2/1, LessThanOrEqual1/1, LessThanOrEqual/1
  Va*/1 -> LessThanOrEqual/2
  Vb*/1 -> LessThanOrEqual1/2
  Vc*/1 -> LessThanOrEqual2/2
  Mux/1 -> Gatings/1
  LessThanOrEqual/1 -> NOT/1, Mux/1
  NOT/1 -> Mux/2
  LessThanOrEqual1/1 -> NOT1/1, Mux/3
  NOT1/1 -> Mux/4
  LessThanOrEqual2/1 -> NOT2/1, Mux/5
  NOT2/1 -> Mux/6

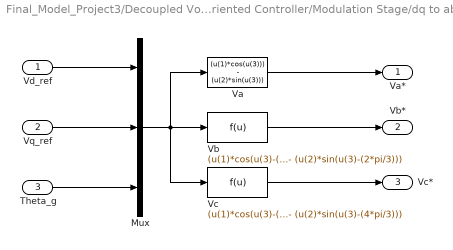
== system Final_Model_Project3/Decoupled Voltage-Oriented Controller/Modulation Stage/dq to abc Transformation ==
  Vd_ref : Inport
  Vq_ref : Inport  Port=2
  Theta_g : Inport  Port=3
  Mux : Mux  Inputs=3
  Va : Fcn  Expr=(u(1)*cos(u(3))) - (u(2)*sin(u(3)))
  Vb : Fcn  Expr=(u(1)*cos(u(3)-(2*pi/3))) - (u(2)*sin(u(3)-(2*pi/3)))
  Vc : Fcn  Expr=(u(1)*cos(u(3)-(4*pi/3))) - (u(2)*sin(u(3)-(4*pi/3)))
  Va* : Outport
  Vb* : Outport  Port=2
  Vc* : Outport  Port=3
  wires:
  Vq_ref/1 -> Mux/2
  Theta_g/1 -> Mux/3
  Vd_ref/1 -> Mux/1
  Va/1 -> Va*/1
  Mux/1 -> Vc/1, Vb/1, Va/1
  Vb/1 -> Vb*/1
  Vc/1 -> Vc*/1

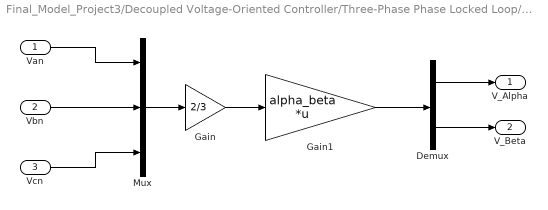
== system Final_Model_Project3/Decoupled Voltage-Oriented Controller/Three-Phase Phase Locked Loop/Alpha - Beta Transformation ==
  Van : Inport
  Vbn : Inport  Port=2
  Vcn : Inport  Port=3
  Demux : Demux  Outputs=2
  Gain : Gain  Gain=2/3
  Gain1 : Gain  Gain=alpha_beta  Multiplication=Matrix(K*u)
  Mux : Mux  Inputs=3
  V_Alpha : Outport
  V_Beta : Outport  Port=2
  wires:
  Vbn/1 -> Mux/2
  Van/1 -> Mux/1
  Vcn/1 -> Mux/3
  Mux/1 -> Gain/1
  Gain/1 -> Gain1/1
  Gain1/1 -> Demux/1
  Demux/1 -> V_Alpha/1
  Demux/2 -> V_Beta/1

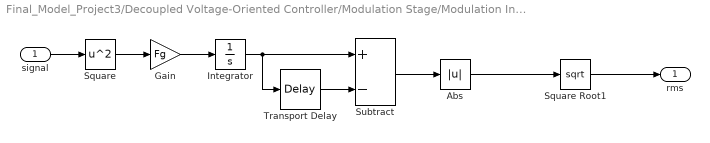
== system Final_Model_Project3/Decoupled Voltage-Oriented Controller/Modulation Stage/Modulation Index Calculation/RMS ==
  signal : Inport
  Abs : Abs  SaturateOnIntegerOverflow=off
  Gain : Gain  Gain=Fg
  Integrator : Integrator
  Square : Math  Operator=square
  Square Root1 : Sqrt
  Subtract : Sum  Inputs=+-
  Transport Delay : TransportDelay  DelayTime=1/Fg
  rms : Outport
  wires:
  signal/1 -> Square/1
  Square/1 -> Gain/1
  Gain/1 -> Integrator/1
  Integrator/1 -> Transport Delay/1, Subtract/1
  Transport Delay/1 -> Subtract/2
  Subtract/1 -> Abs/1
  Abs/1 -> Square Root1/1
  Square Root1/1 -> rms/1
